simulink subsystem "PvtSubSys_LATC"  (R2020b)
settings: Solver=VariableStepAuto  StartTime=0.0  StopTime=10.0  RelTol=1e-3
undefined symbols (not defined in the file or in its folder): LCS_PLAN_PreViewIdxNum, LCS_PLAN_PreViewIdxSW_b, P_Global_CharSpd_ms, P_Global_SteeringAngleRatio, P_Global_WheelBase_m, P_LCS_DetNoOverRide_DrvTrq_TH, P_LCS_DetOverRide_DrvTrq_TH, P_LCS_ESS_AngleSlope_Limit, P_LCS_ESS_LogicTest_Enable, P_LCS_ESS_NotActiveFlgDelayTime, P_LCS_ESS_NotActiveFlgDelayTimeSW, P_LCS_ESS_SteerAngleErr, P_LCS_ESS_SteerAngleFilterTime, P_LCS_ESS_TarAngleFilterTime, P_LCS_ESSAngleSW, P_LCS_ESSOverrideTime1, P_LCS_ESSOverrideTime2, P_LCS_ESSOverrideTime3, P_LCS_ESSOverrideValue1, P_LCS_ESSOverrideValue2, P_LCS_IN_Offset_Test_SW, P_LCS_IN_Offset_Test_Value, P_LCS_LATC_AngleFilterTime_s, P_LCS_LATC_CurOffsetA2FliterT_s, P_LCS_LATC_CurOffsetCurve_TabX_m, P_LCS_LATC_CurOffsetCurveFliterTime_Tab_s, P_LCS_LATC_CurOffsetVehicleSpdLimitValue_degs, P_LCS_LATC_DeltaEps_Tab_s, P_LCS_LATC_DxOffset_Sw, P_LCS_LATC_ELKAngleSlope_ratio, P_LCS_LATC_ELKMaxLatAcc_ms2, P_LCS_LATC_ESSA0Dis_TabX_m, P_LCS_LATC_ESSAddAngleSlope_Tab_degs, P_LCS_LATC_ESSAESAngleSlope_Tab_degs, P_LCS_LATC_ESSAngleSlope_ratio, P_LCS_LATC_ESSMaxLatAcc_ms2, P_LCS_LATC_LCAngleSlope_ratio, P_LCS_LATC_LCAngleSlope_Tab_degs, P_LCS_LATC_LCCancleMaxLatAcc_ms2, P_LCS_LATC_LCEcoAngleSlope_ratio, P_LCS_LATC_LCEcoAngleSlope_Tab_degs, P_LCS_LATC_LCEcoMaxLatAcc_ms2, P_LCS_LATC_LCKAngleSlope_ratio, P_LCS_LATC_LCKAngleSlope_Tab_degs, P_LCS_LATC_LCKIEAngleSlope_ratio, P_LCS_LATC_LCKIEAngleSlope_Tab_degs, P_LCS_LATC_LCKIEMaxLatAcc_ms2, P_LCS_LATC_LCKMaxLatAcc_ms2, P_LCS_LATC_LCNormalAngleSlope_ratio, P_LCS_LATC_LCNormalAngleSlope_Tab_degs, P_LCS_LATC_LCNormalMaxLatAcc_ms2, P_LCS_LATC_LCSportAngleSlope_ratio, P_LCS_LATC_LCSportAngleSlope_Tab_degs, P_LCS_LATC_LCSportMaxLatAcc_ms2, P_LCS_LATC_LKAAngleSlope_ratio, P_LCS_LATC_LKAAngleSlope_Tab_degs, P_LCS_LATC_LKAMaxLatAcc_ms2, P_LCS_LATC_MatrixQ1_st, P_LCS_LATC_MatrixQ3_st, P_LCS_LATC_MatrixR_st ... (+77)
libraries: simulink x38
(part 6 of 7)

== matlab function PvtSubSys_LATC/LATC/LateralControl/LCS_Angle/Motion_Planning/CartesianTrajectory_MPC/CartesianTrajectory ==
  data: planX output single size=11; planY output single size=11; vEgo input size=1; planValid output boolean size=1; kapEgo input size=1; axEgo input size=1; TarLineValid input boolean size=1; TarLineC3 input size=1; TarLineC2 input size=1; TarLineC1 input size=1; TarLineC0 input size=1; ayDtLimit input size=1; planT output; LoopNum output; planLength output; Ay output size=11; AyDt output size=11; break_Flg output; break_AyValue output; break_AyDtValue output; PreDis input; Dis_Fac input; Min_PlanDis input
function [planX,planY,planValid,planT,LoopNum,planLength,Ay,AyDt,break_Flg,break_AyValue,break_AyDtValue] = ...
    linePlanCalc(vEgo, kapEgo,axEgo,...
    TarLineValid,TarLineC3,TarLineC2,TarLineC1,TarLineC0,...
    ayDtLimit,PreDis,Dis_Fac,Min_PlanDis)
%五次多项式规划
LoopNum = 0;
if TarLineValid
    if (abs(TarLineC0)<single(0)) && (abs(TarLineC1)<single(0.05))  %控制线不走中心线，走规划线
        planValid = true;
        planT = single(11);
        planX = single(zeros(11,1));
        planY = single(zeros(11,1));
        planX = single((linspace(0,40,11)))';
        planY = TarLineC3.*planX.^3 + TarLineC2.*planX.^2 + TarLineC1*planX + TarLineC0;
        planLength = planX(end,1);
        Ay = single(zeros(11,1));
        AyDt = single(zeros(11,1));
        break_Flg = uint8(0);
        break_AyValue = single(0);
        break_AyDtValue = single(0);
    else
        Px =single([1.4 1.6 2.1 2.3 2.5 2.7 3 3.3 3.6 4 4.4 4.8 5.3 5.8 6.4 7.1 7.8 8.6 9.5 10.4 11.4]);% 按等比1.1  初选规划时间
        % 定义 TarEgoV、TarEgoAx，由于时间点数变化，导致轨迹条数变化，因此TarEgoV、TarEgoAx维数需要重新定义
        TarEgoAx = zeros(1,length(Px));
        TarEgoV = ones(1,length(Px)) .* vEgo;
        
        if vEgo>single(1)
            Px = vEgo*Px;   %纵向行驶距离
        end
        
        Py = TarLineC3*(Px.^3) + TarLineC2*(Px.^2) + TarLineC1*(Px.^1) + TarLineC0;
        x = single(zeros(11,1));
        y = single(zeros(11,1));
        Vx = single(zeros(11,1));
        Vy = single(zeros(11,1));
        Ax = single(zeros(11,1));
        Ay = single(zeros(11,1));
        AyDt = single(zeros(11,1));
        
        break_Flg = uint8(0);
        break_AyValue = single(0);
        break_AyDtValue = single(0);

        Pt = single(zeros(1,1));  
        for i = 1:length(Px)   
            Pt = 1.05*sqrt(Px(i)^2 + Py(i)^2)/max(1,0.5*(TarEgoV(i) + vEgo));  %规划时间
            t_Vego = max(vEgo,1);
            t0 = single(0);
            tn = Pt;
            
            T = [t0^5,t0^4,t0^3,t0^2,t0,1;...
                5*t0^4,4*t0^3,3*t0^2,2*t0,1,0;...
                20*t0^3,12*t0^2,6*t0,2,0,0;...
                tn^5,tn^4,tn^3,tn^2,tn,1;...
                5*tn^4,4*tn^3,3*tn^2,2*tn,1,0;...
                20*tn^3,12*tn^2,6*tn,2,0,0];    
            
            Vn = TarEgoV(i);
            An = TarEgoAx(i);
            kP =  3*TarLineC3*(Px(i).^2) + 2*TarLineC2*Px(i) + TarLineC1;  %规划线的斜率
            
            Kap = 6*TarLineC3*(Px(i))+2*TarLineC2;      
            Arcf = (vEgo^2)*Kap;                          
            Ayn = Arcf/sqrt(1 + kP^2);                       
            Axn = Arcf*kP/sqrt(1 + kP^2);                              
            Vxn = Vn/sqrt(1 + kP^2);                         
            Vyn = Vn*kP/sqrt(1 + kP^2);
            
            MaX = [0;t_Vego;axEgo;Px(i);Vxn;Axn];            
            MaY = [0;0;(vEgo^2)*kapEgo;Py(i);Vyn;Ayn];
            %求解多项式
            A = T\MaX;
            B = T\MaY;
            
            a5 = A(1);
            a4 = A(2);
            a3 = A(3);
            a2 = A(4);
            a1 = A(5);
            a0 = A(6);
            
            b5 = B(1);
            b4 = B(2);
            b3 = B(3);
            b2 = B(4);
            b1 = B(5);
            b0 = B(6);
            
            preLineValid = true;
            for j=1:11
                t = (j-1)*tn/10;
                x(j) = a5*t^5 + a4*t^4 + a3*t^3 + a2*t^2 + a1*t + a0;
                Vx(j) = 5*a5*t^4 + 4*a4*t^3 + 3*a3*t^2 + 2*a2*t + a1;
                Ax(j) = 20*a5*t^3 + 12*a4*t^2 + 6*a3*t + 2*a2;
                y(j) = b5*t^5 + b4*t^4 + b3*t^3 + b2*t^2 + b1*t + b0;
                Vy(j) = 5*b5*t^4 + 4*b4*t^3 + 3*b3*t^2 + 2*b2*t + b1;
                Ay(j) = 20*b5*t^3 + 12*b4*t^2 + 6*b3*t + 2*b2;
                AyDt(j) = 60*b5*t^2 + 24*b4*t + 6*b3;

                if (abs(AyDt(j))>ayDtLimit)
                    break_Flg = uint8(1);
                    break_AyValue = abs(Ay(j));
                    break_AyDtValue = abs(AyDt(j));
                    preLineValid = false;
                    break;
                end
            end
            if ((sqrt(x(11)^2 + y(11)^2)) < Min_PlanDis) || ((sqrt(x(11)^2 + y(11)^2))*Dis_Fac < (PreDis + 2.1))
                preLineValid = false;
            end
            if preLineValid
                break_Flg = uint8(3);
                break_AyValue = max(abs(Ay));
                break_AyDtValue = max(abs(AyDt(j)));
                break;
            end
            
            if i == length(Px) % 此处存在都不满足的情况，需要按最长时间输出。经测试发现如果按最长时间输出会控不住车辆。暂时改成跟随目标线
                planValid = true;
                Pt = single(Px(i));
                x = single(zeros(11,1));
                y = single(zeros(11,1));
                x = single((linspace(0,40,11)))';
                y = TarLineC3.*x.^3 + TarLineC2.*x.^2 + TarLineC1*x + TarLineC0;
                break_Flg = uint8(4);
                break_AyValue = single(0);
                break_AyDtValue = single(0);
            end
        end
        LoopNum = i;
        planValid = true;
        planT = Pt;
        planX = x;
        planY = y;
        planLength = planX(end,1);
    end
else
    planValid = false;
    planT = single(0);
    planX = single(zeros(11,1));
    planY = single(zeros(11,1));
    LoopNum = 0;
    planLength = planX(end,1);
    Ay = single(zeros(11,1));
    AyDt = single(zeros(11,1));
    break_Flg = uint8(0);
    break_AyValue = single(0);
    break_AyDtValue = single(0);
end

== matlab function PvtSubSys_LATC/LATC/LateralControl/LCS_Angle/Motion_Planning/FrenetTrajectory/Subsystem/MATLAB Function1 ==
  data: Delaytime input uint16; Flg output uint8; Count output uint16; TarDangerLevel input uint8; TarDangerLevelK1 input uint8; FlgK1 input uint8; CountK1 input uint16
function [Flg,Count]= fcn(Delaytime,TarDangerLevel,TarDangerLevelK1,FlgK1,CountK1)
Count = min(CountK1 + uint16(1),Delaytime);
if Count == Delaytime
    Flg = uint8(0);
else
    Flg = FlgK1;
end
%%状态检测
if TarDangerLevel == uint8(1) && TarDangerLevelK1 == 0 %功能激活
    Count = uint16(0);
    Flg = uint8(1);  
end
end

== matlab function PvtSubSys_LATC/LATC/LateralControl/EPSFaultCheck/MATLAB Function1 ==
  data: u input; y output uint8; countK input uint8; count output uint8
function [y,count] = fcn(u,countK)
count = countK - uint8(1);
if u>0
    count = uint8(3000);
end
if count > 1
    y = uint8(0);
else
    y = uint8(1);
end

== matlab function PvtSubSys_LATC/LATC/LateralControl/LCS_Angle/Lateral_Control/Dynamic_Model_LQR/TarSteerAngleCalc ==
  data: steer_angle_cmd_temp output; steer_feedforward_temp output; steer_feedbackward_temp output; steer_limit_temp output; LineValid input; SteerAngle input; steer_angle output size=[1,1]; Veh_Speed input; ref_curvature input; lateral_error input; lateral_error_rate input; heading_error input; heading_error_rate input; Left_steer_ratio input; Right_steer_ratio input; Matrix_q1 input; Matrix_q3 input; Matrix_R input; Max_lateral_acceleration input; TarSteerAngleSlope input; CurrentSteerAngleOffset input; steer_angleK1 input single
function [steer_angle_cmd_temp,steer_feedforward_temp,steer_feedbackward_temp,steer_limit_temp,steer_angle]= LQR_Algorithm(LineValid,SteerAngle,Veh_Speed,ref_curvature,lateral_error,lateral_error_rate,heading_error,heading_error_rate,...
    Left_steer_ratio,Right_steer_ratio,Matrix_q1,Matrix_q3,Matrix_R,Max_lateral_acceleration,TarSteerAngleSlope,CurrentSteerAngleOffset,steer_angleK1)
if LineValid
    %% 1.车辆参数
    %1.1 车的大小及长度参数
    veh_params.vehicle_length = single(4.875);
    veh_params.vehicle_width  = single(2.2);
    veh_params.vehicle_height = single(1.69);
    %1.2 车辆控制参数
    veh_params.wheel_base = single(2.92);               %轴距, m
    veh_params.Vch = single(23.5);                      %特征车速
    veh_params.max_steer_angle = single(53 / 180 * pi); %前轮最大转角
    veh_params.max_acceleration = single(2);            %车辆最大加速度
    veh_params.max_deceleration = single(-2);           %车辆最大减速度
    veh_params.left_steer_ratio = Left_steer_ratio;     %车辆左侧转向传动比%
    veh_params.right_steer_ratio = Right_steer_ratio;   %车辆右侧转向传动比%
    veh_params.cf = single(155494.663);                 %车辆前轮侧偏刚度
    veh_params.cr = single(155494.663);                 %车辆后轮侧偏刚度 
    veh_params.mass_fl = single(520);                   %车辆左前轮负重
    veh_params.mass_fr = single(520);                   %车辆右前轮负重
    veh_params.mass_rl = single(520);                   %车辆左后轮负重
    veh_params.mass_rr = single(520);                   %车辆右后轮负重
    %% 2.控制参数计算
    mass_front =  veh_params.mass_fl + veh_params.mass_fr;     %前轮负载
    mass_rear  =  veh_params.mass_rl + veh_params.mass_rr;     %后轮负载
    mass =  mass_front + mass_rear;                            %这个整车负载  不是整车质量？？？？？？？
    lf = veh_params.wheel_base * (single(1.0) - mass_front / mass);
    lr = veh_params.wheel_base * (single(1.0) - mass_rear / mass);
    iz = lf * lf * mass_front + lr * lr * mass_rear;
    %% 3.LQR参数设置
    
    lqr_eps = single(0.01);    %最小精度
    lqr_max_iteration = single(800);    %最大迭代次数
    
    basic_state_size = uint8(4);     
    control_size = uint8(1);
    
    matrix_a = single(zeros(basic_state_size,basic_state_size));
    matrix_a_coeff = single(zeros(basic_state_size,basic_state_size));
    I = single(eye(basic_state_size,basic_state_size));
    matrix_a(1,2) = single(1.0);
    matrix_a(2,3) = single((veh_params.cf + veh_params.cr ) / mass);
    matrix_a(3,4) = single(1.0);
    matrix_a(4,3) = single((lf * veh_params.cf - lr * veh_params.cr) / iz);
    
    matrix_a_coeff(2,2) = single(-(veh_params.cf + veh_params.cr) / mass);
    matrix_a_coeff(2,4) = single((lr * veh_params.cr - lf * veh_params.cf) / mass);
    matrix_a_coeff(3,4) = single(1.0);
    matrix_a_coeff(4,2) = single((lr * veh_params.cr - lf * veh_params.cf) / iz);
    matrix_a_coeff(4,4) = single(-1.0 * (lf * lf * veh_params.cf + lr * lr * veh_params.cr)/iz);
    
    matrix_a(2,2) = matrix_a_coeff(2,2);
    matrix_a(2,4) = matrix_a_coeff(2,4);
    matrix_a(4,2) = matrix_a_coeff(4,2);
    matrix_a(4,4) = matrix_a_coeff(4,4);
    
    matrix_b = single(zeros(basic_state_size,control_size));
    matrix_b(2,1) = veh_params.cf/mass;
    matrix_b(4,1) = lf * veh_params.cf /iz;
    
    matrix_q = single(zeros(4,4));
    matrix_q(1,1) = Matrix_q1;                      %调整q矩阵的第一、三个参数，改善转向性能0.0001,0.02  Q为状态权重系数
    matrix_q(3,3) = Matrix_q3;
    matrix_r = single(zeros(1,1));
    matrix_r = Matrix_R;                            %R为控制量权重系数
    
    lqr_params.A = matrix_a;
    lqr_params.B = matrix_b;
    lqr_params.I = I;
    lqr_params.ts = single(0.02);
    lqr_params.lr = lr;
    lqr_params.lf = lf;
    lqr_params.cf=veh_params.cf;
    lqr_params.cr=veh_params.cf;
    lqr_params.iz=iz;
    lqr_params.mass=mass;
    lqr_params.Q =matrix_q ;
    lqr_params.R = matrix_r;
    lqr_params.eps=lqr_eps;
    lqr_params.max_iteration=lqr_max_iteration;
    %% 4.计算前轮转角
    lqr_params.A(2,2) = lqr_params.A(2,2)/(max(Veh_Speed, single(0.2)));
    lqr_params.A(2,4) = lqr_params.A(2,4)/(max(Veh_Speed, single(0.2)));
    lqr_params.A(4,2) = lqr_params.A(4,2)/(max(Veh_Speed, single(0.2)));
    lqr_params.A(4,4) = lqr_params.A(4,4)/(max(Veh_Speed, single(0.2)));
    
    A=lqr_params.A;
    B=lqr_params.B;
    I=lqr_params.I;
    ts=lqr_params.ts;      %控制周期
    min_tol = lqr_params.eps;    %0.01  这个时间是什么意思？？？？？？
    max_iter = lqr_params.max_iteration;   %800   这个是什么意思？？？？？
    matrix_Q = lqr_params.Q;
    matrix_R = lqr_params.R;
    
    matrix_ad=single(zeros(size(A)));   %4*4零矩阵
    matrix_ad=(I+ts*single(0.5) * A) / (I-ts*single(0.5) * A);  %离散化 系数 A=(I-TA/2)/(I-TA/2) B=TB
    
    matrix_bd=single(zeros(size(B)));
    matrix_bd=B*ts;
    matrix_k = SolveLQRProblem(matrix_ad, matrix_bd, matrix_Q,matrix_R, min_tol, max_iter);  %求解最优解K
    %% 横向状态变量
    
    matrix_state = single(zeros(4, 1));
    matrix_state(1, 1) = lateral_error;                   %横向误差
    matrix_state(2, 1) = lateral_error_rate;              %横向误差率
    matrix_state(3, 1) = heading_error;                   %航向误差
    matrix_state(4, 1) = heading_error_rate;              %航向误差率
    steer_feedbackward = -(matrix_k * matrix_state);      %反馈控制器
    % 前馈转角
    kv = lqr_params.lr * lqr_params.mass / single(1) / lqr_params.cf / veh_params.wheel_base - ...
        lqr_params.lf * lqr_params.mass / single(1) / lqr_params.cr / veh_params.wheel_base;
    steer_feedforward = (veh_params.wheel_base * ref_curvature + kv * Veh_Speed * Veh_Speed * ref_curvature - matrix_k(1, 3) * ...
        (lqr_params.lr * ref_curvature - lqr_params.lf * lqr_params.mass * Veh_Speed * Veh_Speed * ref_curvature / single(1) / lqr_params.cr / veh_params.wheel_base));%弧度制角度rad
    % 4.3 计算期望前轮偏角
    steer_cmd = steer_feedforward + steer_feedbackward;
    
    if (steer_cmd>=0)
        steer_transmission_ratio = veh_params.left_steer_ratio;
    else
        steer_transmission_ratio = veh_params.right_steer_ratio;
    end
    steer_feedforward_temp = steer_feedforward * single(57.3) * steer_transmission_ratio;%反算方向盘转角并转换为角度制deg
    steer_feedbackward_temp = steer_feedbackward * single(57.3) * steer_transmission_ratio;%反算方向盘转角并转换为角度制deg
    steer_angle_cmd = steer_cmd * single(57.3) * steer_transmission_ratio;%反算方向盘转角并转换为角度制deg
    steer_angle_cmd_temp = steer_angle_cmd;%输出算法计算角度作为观测，最终请求角度会补偿转向不足。
    %% 5.限制期望前轮偏角
    % 5.1 根据横向加速度限制前轮转角
    if Veh_Speed < 1
        steer_limit = atan( Max_lateral_acceleration * veh_params.wheel_base /(Veh_Speed *Veh_Speed))* single(57.3) * steer_transmission_ratio; % 高速计算不准确，更改为下面特征车速计算方法
    else
        AckConst = min((single(1)+Veh_Speed*Veh_Speed/(veh_params.Vch*veh_params.Vch))*veh_params.wheel_base/max(single(1),Veh_Speed),single(32767));
        % PsiDtAckRaw = (SteerAngle/steer_transmission_ratio)/AckConst;
        steer_limit = ((Max_lateral_acceleration * AckConst)/Veh_Speed)* single(57.3) * steer_transmission_ratio;
    end
    %     steer_limit = atan( Max_lateral_acceleration * veh_params.wheel_base /(Veh_Speed *Veh_Speed)) * steer_transmission_ratio;
    steer_angle_cmd = min(steer_limit, max(-steer_limit,steer_angle_cmd));%方向盘角度制deg
    
    steer_angle_deg = steer_angle_cmd + CurrentSteerAngleOffset;
    steer_limit_temp = steer_limit;
    % 5.2 限制方向盘转速
    steer_angle = min(steer_angleK1 + TarSteerAngleSlope,max(steer_angleK1 - TarSteerAngleSlope,steer_angle_deg));
    
else
    steer_angle = SteerAngle;
    steer_angle_cmd_temp = single(0);
    steer_feedforward_temp = single(0);
    steer_feedbackward_temp = single(0);
    steer_limit_temp = single(0);
end
end

== matlab function PvtSubSys_LATC/LATC/LateralControl/LCS_Angle/Motion_Planning/CartesianTrajectory/Subsystem1/MATLAB Function ==
  data: Forward_PreViewT input; VehSpd input; PreCurve output; C2 input; C3 input; PreCurve_Abs output
function [PreCurve,PreCurve_Abs]= PreView_Point_Curvature(Forward_PreViewT,VehSpd,C2,C3)
LookForwardDis = VehSpd * Forward_PreViewT;
PreCurve = 6*C3*LookForwardDis + 2*C2;
PreCurve_Abs = abs(PreCurve);
end

== matlab function PvtSubSys_LATC/LATC/LateralControl/LCS_Angle/Motion_Planning/CartesianTrajectory/Subsystem1/MATLAB Function1 ==
  data: Delaytime input uint16; Flg output uint8; Count output uint16; TarDangerLevel input uint8; TarDangerLevelK1 input uint8; FlgK1 input uint8; CountK1 input uint16
function [Flg,Count]= fcn(Delaytime,TarDangerLevel,TarDangerLevelK1,FlgK1,CountK1)
Count = min(CountK1 + uint16(1),Delaytime);
if Count == Delaytime
    Flg = uint8(0);
else
    Flg = FlgK1;
end
%%状态检测
if TarDangerLevel == uint8(1) && TarDangerLevelK1 == 0 %功能激活
    Count = uint16(0);
    Flg = uint8(1);  
end
end

== matlab function PvtSubSys_LATC/LATC/LateralControl/LCS_Angle/Motion_Planning/CartesianTrajectory/FrenetTrajectory ==
  data: A0 input; A1 input; A2 input; A3 input; Veh_Speed input size=1; YawRate input size=1; PreView_T input size=1; PlanX output; PlanY output; PlanTheta output; idx output; PreviewX output; PreviewY output; PreviewTheta output; numTraj output size=1; ref_curvature output; ref_theta output; AyDtLimit input size=1; Min_Plan_Dis input; lateral_error output size=1; lateral_error_rate output size=1; heading_error output size=1; heading_error_rate output size=1; axEgo input; kapEgo input; PreViewIdxSW input size=[1,1]; PreViewIdxNum input size=[1,1]
function [PlanX,PlanY,PlanTheta,idx,PreviewX,PreviewY,PreviewTheta,numTraj,ref_curvature,ref_theta,lateral_error,lateral_error_rate,heading_error,heading_error_rate] ...
    = FrenetTrajectory(A0,A1,A2,A3,Veh_Speed,YawRate,PreView_T,AyDtLimit,Min_Plan_Dis,axEgo,kapEgo,PreViewIdxSW,PreViewIdxNum)
%% 生成轨迹
Px =single([1.5 2 2.5 2.7 3 3.3 3.6 4 4.4 4.8 5.3 5.8 6.4 7.1 7.8 8.6 9.5 10.4 11.4]); %Py_Fac后期去掉，增加一个轨迹筛选条件，每个车速下最小规划距离
TarEgoAx = zeros(1,length(Px));   %初始化矩阵
TarEgoV = ones(1,length(Px)) .* Veh_Speed;  %计算纵向行驶距离
if Veh_Speed>single(1)
    Px = Veh_Speed*Px;    %纵向距离 l 
end 
Py = A3*(Px.^3) + A2*(Px.^2) + A1*(Px.^1) + A0;  
x = single(zeros(11,1));
y = single(zeros(11,1));
Vx = single(zeros(11,1));
Vy = single(zeros(11,1));
Ax = single(zeros(11,1));
Ay = single(zeros(11,1));
AyDt = single(zeros(11,1));
Pt = single(zeros(1,1));     %规划时间
for i = 1:length(Py)
    Pt = 1.05*sqrt(Px(i)^2 + Py(i)^2)/max(1,0.5*(TarEgoV(i) + Veh_Speed));   
    t_Vego = max(Veh_Speed,1);
    t0 = single(0);
    tn = Pt;
    T = [t0^5,t0^4,t0^3,t0^2,t0,1;...
        5*t0^4,4*t0^3,3*t0^2,2*t0,1,0;...
        20*t0^3,12*t0^2,6*t0,2,0,0;...
        tn^5,tn^4,tn^3,tn^2,tn,1;...
        5*tn^4,4*tn^3,3*tn^2,2*tn,1,0;...
        20*tn^3,12*tn^2,6*tn,2,0,0];
    Vn = TarEgoV(i);
    An = TarEgoAx(i);
    kP =  3*A3*(Px(i).^2) + 2*A2*Px(i) + A1;
    
    Kap = 6*A3*(Px(i))+2*A2;
    Arcf = (Veh_Speed^2)*Kap;
    Ayn = Arcf/sqrt(1 + kP^2);
    Axn = Arcf*kP/sqrt(1 + kP^2);
    
    Vxn = Vn/sqrt(1 + kP^2);
    Vyn = Vn*kP/sqrt(1 + kP^2);
    MaX = [0;t_Vego;axEgo;Px(i);Vxn;Axn];
    MaY = [0;0;(Veh_Speed^2)*kapEgo;Py(i);Vyn;Ayn];
    A = T\MaX;
    B = T\MaY;
    
    a5 = A(1); % 纵向轨迹系数
    a4 = A(2);
    a3 = A(3);
    a2 = A(4);
    a1 = A(5);
    a0 = A(6);
    
    b5 = B(1); % 横向轨迹系数
    b4 = B(2);
    b3 = B(3);
    b2 = B(4);
    b1 = B(5);
    b0 = B(6);
    preLineValid = true;
    for j=1:11
        t = (j-1)*tn/10;
        x(j) = a5*t^5 + a4*t^4 + a3*t^3 + a2*t^2 + a1*t + a0;
        Vx(j) = 5*a5*t^4 + 4*a4*t^3 + 3*a3*t^2 + 2*a2*t + a1;
        Ax(j) = 20*a5*t^3 + 12*a4*t^2 + 6*a3*t + 2*a2;
        y(j) = b5*t^5 + b4*t^4 + b3*t^3 + b2*t^2 + b1*t + b0;
        Vy(j) = 5*b5*t^4 + 4*b4*t^3 + 3*b3*t^2 + 2*b2*t + b1;
        Ay(j) = 20*b5*t^3 + 12*b4*t^2 + 6*b3*t + 2*b2;
        AyDt(j) = 60*b5*t^2 + 24*b4*t + 6*b3;
        if abs(AyDt(j))>AyDtLimit 
            preLineValid = false;
            break;
        end     
    end
    if abs(sqrt(x(11)^2+y(11)^2)) < Min_Plan_Dis       %规划的距离最小不能小于设定的阈值
       preLineValid = false; 
    end
    if preLineValid
        break;
    end
end
NumTarpoints = 40;       %轨迹点的个数
y = y.*single(-1);
objSpline = Spline2D(y,x);
s = single(linspace(0,objSpline.s(end),NumTarpoints));
TargetPoints = single(zeros(length(s),6));
%% 为什么要转一下直角坐标？？？？？

for i = single(1):single(1):length(s)
    [ix,iy] = objSpline.calc_position(s(i));     %车体坐标转换为直角坐标
    TargetPoints(i,1) = ix;                      %直角坐标中的X 左负右正   车辆横向位置
    TargetPoints(i,2) = iy;                      %直角坐标Y    车辆纵向位置
    TargetPoints(i,3) = objSpline.calc_yaw(s(i));   %车辆Yaw角  横摆角
    TargetPoints(i,4) = objSpline.calc_curvature(s(i));    %曲率
    TargetPoints(i,5) = objSpline.calc_curvatureDerivative(s(i));   %曲率变化率
    TargetPoints(i,6) = s(i);                                  
end
traj = single(zeros(NumTarpoints,6)); t= single(zeros(NumTarpoints,1)); costs = single(zeros(1,1));
globalTrajectory = repmat(struct('Trajectory',traj,'Times',t,'costs',costs), 1, 1);
globalTrajectory(1).Trajectory = TargetPoints;
globalTrajectory(1).Times = t;

numTraj  = i;%借用numTraj输出时间点索引号
%% 直角坐标转换为车体坐标     
% [s,d]→[x, y, theta, kappa, dkappa]
PlanX= globalTrajectory(1).Trajectory(1:NumTarpoints,2);
PlanY= (globalTrajectory(1).Trajectory(1:NumTarpoints,1))*single(-1);
PlanTheta = globalTrajectory(1).Trajectory(1:NumTarpoints,3);
[matrix_state,ref_curvature,ref_theta,idx] = Calc_State_Error(Veh_Speed,YawRate,globalTrajectory,PreView_T,NumTarpoints,PreViewIdxSW,PreViewIdxNum);
PreviewX = globalTrajectory(1).Trajectory(idx,2);
PreviewY = (globalTrajectory(1).Trajectory(idx,1))*single(-1);
PreviewTheta = globalTrajectory(1).Trajectory(idx,3);
% lateral_error = single(zeros(1,1));lateral_error_rate = single(zeros(1,1));heading_error = single(zeros(1,1));heading_error_rate = single(zeros(1,1));
lateral_error = matrix_state(1,1);
lateral_error_rate = matrix_state(2,1);
heading_error = matrix_state(3,1);
heading_error_rate = matrix_state(4,1);

end

== matlab function PvtSubSys_LATC/LATC/LateralControl/ESS_SteerSpd_Test/NotActiveFlgDelayTime/MATLAB Function ==
  data: FlgIn input boolean; FlgOut output boolean size=1; t_offset input single; tcycle input single; FlgOutK1 input boolean; delaytimeK1 input single; delaytime output single size=1; flgK1 input uint8; flg output uint8 size=1
function [FlgOut,delaytime,flg]= fcn(FlgIn,t_offset,tcycle,FlgOutK1,delaytimeK1,flgK1)
FlgOut = FlgIn;
delaytime = single(0);
flg = uint8(0);
if FlgOutK1 ==0 && FlgOut == 1
    flg = uint8(1);
    FlgOut = true;
    delaytime = tcycle;
end
if  flgK1 == 1
     delaytime = delaytimeK1 + tcycle;
      if delaytime < t_offset
          flg = uint8(1);
          FlgOut = true;
      end
end

== matlab function PvtSubSys_LATC/LATC/LateralControl/LCS_Angle/Lateral_Control/kinematics_MPC/SteerAngSlopeCalc/MATLAB Function3 ==
  data: delytime input uint16; TarDangerLevel input uint8; TarDangerLevelK1 input uint8; FLg output uint8; FLgK1 input uint8; CntK1 input uint16; Cnt output uint16
function [FLg,Cnt] = AngSlopeCalc(delytime,TarDangerLevel,TarDangerLevelK1,FLgK1,CntK1)

Cnt = min(CntK1 + uint16(1),delytime);
if Cnt== delytime
    FLg = uint8(0);
else
    FLg = FLgK1;
end
%FLg = FLgK1;
%% 
if TarDangerLevel==uint8(1) && TarDangerLevelK1==0  % NO function 2 LCK (TarDangerLevelK1==0)
    Cnt =uint16(0);
    FLg = uint8(1);
end

if  TarDangerLevel==uint8(3) && (TarDangerLevelK1==uint8(1)||TarDangerLevelK1==uint8(2)) % LCK/IE 2 LC_Normal
    Cnt =uint16(0);
    FLg = uint8(2);
end

if  TarDangerLevel==uint8(7) && (TarDangerLevelK1==uint8(1)||TarDangerLevelK1==uint8(2)) % LCK/IE 2 LC_Eco
    Cnt =uint16(0);
    FLg = uint8(3);
end

if  TarDangerLevel==uint8(8) && (TarDangerLevelK1==uint8(1)||TarDangerLevelK1==uint8(2)) % LCK/IE 2 LC_sport
    Cnt =uint16(0);
    FLg = uint8(4);
end
if  TarDangerLevel==uint8(6) && (TarDangerLevelK1==uint8(1)||TarDangerLevelK1==uint8(2)) % LCK/IE 2 ESS 后期添加配和ESS Slope 一起调试
    Cnt =uint16(0);
    FLg = uint8(5);
end

== matlab function PvtSubSys_LATC/LATC/LateralControl/LCS_Angle/Lateral_Control/kinematics_MPC/TarSteerAngleCalc ==
  data: steer_angle_cmd_temp output; steer_feedforward_temp output; steer_feedbackward_temp output; steer_limit_temp output; matrix_result output; LineValid input; SteerAngle input; steer_angle output size=[1,1]; Veh_Speed input; ref_curve input; ref_theta input; Delta_t input; lateral_error input; heading_error input; Umax input; Delta_umax input; Left_steer_ratio input; Right_steer_ratio input; Matrix_q1 input; Matrix_q2 input; Matrix_r input; Max_lateral_acceleration input; TarSteerAngleSlope input; CurrentSteerAngleOffset input; steer_angleK1 input single; U_k output; U_k1 input single
function [steer_angle_cmd_temp,steer_feedforward_temp,steer_feedbackward_temp,steer_limit_temp,matrix_result,steer_angle,U_k]= ...
    kinematics_MPC(LineValid,SteerAngle,Veh_Speed,ref_curve,ref_theta,Delta_t,lateral_error,heading_error,Umax,Delta_umax,...
    Left_steer_ratio,Right_steer_ratio,Matrix_q1,Matrix_q2,Matrix_r,Max_lateral_acceleration,TarSteerAngleSlope,CurrentSteerAngleOffset,steer_angleK1,U_k1)
if LineValid
    %% 1.车辆参数
    %1.1 车的大小及长度参数
    veh_params.vehicle_length = single(4.875);
    veh_params.vehicle_width  = single(2.2);
    veh_params.vehicle_height = single(1.69);
    %1.2 车辆控制参数
    veh_params.wheel_base = single(2.92);               %轴距, m
    veh_params.Vch = single(23.5);                      %特征车速
    veh_params.max_steer_angle = single(53 / 180 * pi); %前轮最大转角  
    veh_params.max_acceleration = single(2);            %车辆最大加速度
    veh_params.max_deceleration = single(-2);           %车辆最大减速度
    veh_params.left_steer_ratio = Left_steer_ratio;     %车辆左侧转向传动比%
    veh_params.right_steer_ratio = Right_steer_ratio;   %车辆右侧转向传动比%
    veh_params.cf = single(155494.663);                 %车辆前轮侧偏刚度
    veh_params.cr = single(155494.663);                 %车辆后轮侧偏刚度 
    veh_params.mass_fl = single(520);                   %车辆左前轮负重
    veh_params.mass_fr = single(520);                   %车辆右前轮负重
    veh_params.mass_rl = single(520);                   %车辆左后轮负重
    veh_params.mass_rr = single(520);                   %车辆右后轮负重
    %% 2.控制参数计算
    %% 3.MPC矩阵
    Np = single(10);
    Nc = single(5);
    Row = single(10); %松弛因子
    ref_delta = atan(veh_params.wheel_base * ref_curve);   %前轮转角
    %% 离散状态空间方程
    A = [ 1  Veh_Speed * cos(ref_theta) * Delta_t;    %一个是航向角一个是前轮转角  这里都用前轮转角对吗？
        0  1 ];
    B = [ 0;
        Veh_Speed * Delta_t / (veh_params.wheel_base * cos(ref_delta)^2)];
    Nx = size(A,1); %状态量个数 2 横向车速V及航向角
    Nu = size(B,2); %控制量个数 1 前轮转角
    % 对状态量进行增广
    kesi = zeros(Nx,Nu); % 构造新的状态量矩阵   2*1
    kesi = cat(1,kesi,U_k1);% 将上一时刻的前轮偏角误差放在第3行，进行状态增广3*1维矩阵
    kesi(1) = lateral_error;
    kesi(2) = lateral_error;  %即kesi矩阵为[lateral_error;lateral_error;ref_delta_error]
    %% 定义Q R矩阵
    matrix_q = [Matrix_q1 0;
                0 Matrix_q2];
    matrix_r = Matrix_r;
    matrix_Q = zeros(Np*Nx,Np*Nx);%20*20
    matrix_Q_temp = zeros(Nx,Np*Nx);%2*20
    for i=1:Np
        for j= 1:Np
            if i == j
                matrix_Q_temp = zeros(Nx,Np*Nx);
                matrix_Q_temp(:,((j-1)*Nx+1):j*Nx) = matrix_q;
            end
        end
        matrix_Q(((i-1)*Nx+1):i*Nx,:) = matrix_Q_temp;
    end
    matrix_R = zeros(Nc*Nu,Nc*Nu);%10*10
    matrix_R_temp = zeros(Nu,Nc*Nu);
    for i=1:Nc
        for j= 1:Nc
            if i == j
                matrix_R_temp = zeros(Nu,Nc*Nu);
                matrix_R_temp(:,((j-1)*Nu+1):j*Nu) = matrix_r;
            end
        end
        matrix_R(((i-1)*Nu+1):i*Nu,:) = matrix_R_temp;
    end
    % 按增量式对矩阵进行增广
    A = [A B;zeros(Nu,Nx) eye(Nu)]; % 3*3
    B = [B;eye(Nu)]; % 3*1
    % 定义输出矩阵
    C = single([1 0 0;0 1 0;]);% 2*3
    % THETA和PHI
    PHI = zeros(Np*Nx,size(A,2));    %20*3
    THETA = zeros(Np*Nx,Nc*Nu);      %20*5
    THETA_temp = zeros(Nx,Nc*Nu);    %2*5
    for r=1:Np
        for c=1:Nc
            if c<=r
                THETA_temp(:,((c-1)*Nu+1):c*Nu)=C*A^(r-c)*B; %2*3*3*3*1
            end
        end
        THETA(((r-1)*Nx+1):r*Nx,:) = THETA_temp;
        PHI(((r-1)*Nx+1):r*Nx,:) =  C*A^r; %2*3*3*3
    end
    
    % 构造二次规划的H矩阵
    H_temp = THETA'*matrix_Q*THETA + matrix_R;
    H = [H_temp zeros(Nu*Nc,1);zeros(1,Nu*Nc) Row];
    H = single(2)*H;
    H = (H+H')/single(2);
    % E矩阵
    error = PHI*kesi; %这里的error就是我们所设的E矩阵
    % f矩阵
    f_temp = single(2)*error'* matrix_Q * THETA;
    f = zeros(size(f_temp,1),(size(f_temp,2)+1));
    f(:,1:size(f_temp,2)) = f_temp;
    %% 约束生成区域
    % 不等式约束
    A_t = tril(ones(Nc,Nc),0);
    A_I=kron(A_t,eye(Nu));
    Ut=kron(ones(Nc,1),U_k1);                 %此处的U表示的应该是上一时刻控制量误差（即偏差）组成的矩阵。
    umin = -Umax/single(57.3);                %维数与控制变量的个数相同
    umax = Umax/single(57.3);                 %此处的最大值最小值约束，是对控制量误差的最大最小值进行约束，此处理解的物理意义是在参考转角上下一个范围内进行约束求解
    
    delta_umin =  -Delta_umax/single(57.3)*Delta_t;
    delta_umax =   Delta_umax/single(57.3)*Delta_t;
    Umin=kron(ones(Nc,1),umin);
    Umax=kron(ones(Nc,1),umax);
%     A_cons = [A_I zeros(Nu*Nc,1);-A_I zeros(Nu*Nc,1)];
%     b_cons = [Umax-Ut;-Umin+Ut];
    % 上下限约束
    EM = single(10);
    delta_Umin=kron(ones(Nc,1),delta_umin);
    delta_Umax=kron(ones(Nc,1),delta_umax);
    lb=[delta_Umin;-EM];%（求解方程）状态量下界，包含控制时域内控制增量和松弛因子下界M
    ub=[delta_Umax;EM];%（求解方程）状态量上界，包含控制时域内控制增量和松弛因子上界M
    % 两种约束合并
    A_cons2 = [A_I zeros(Nu*Nc,1);-A_I zeros(Nu*Nc,1);eye((Nu*Nc)+1);-eye((Nu*Nc)+1)];
    b_cons2 = [Umax-Ut;-Umin+Ut;ub;-lb];
    %% 二次规划求解
    % Format in qp_solver
    % min 0.5*x'*H*x + f'*x   subject to:  A*x <= b
    % with respect to:  A * x = b (equality constraint)
    % A*x <= b (inequality constraint)
    % solve QR problem
    % [matrix_result] = mpcCustomSolverCodeGen(single(H),single(f), single(-A_cons2), single(-b_cons2));
    matrix_result = single(zeros(Nc+1,1));
    matrix_result = MPC_Solver_QPhild(H,f',A_cons2,b_cons2);
    %% 4.计算前轮转角
    u_piao = matrix_result(1);
    U_k = single(kesi(3)) + u_piao;
    steer_cmd = ref_delta + U_k;
    %% 反算方向盘转角并转换为角度制
    if (steer_cmd>=0)
        steer_transmission_ratio = veh_params.left_steer_ratio;
    else
        steer_transmission_ratio = veh_params.right_steer_ratio;
    end
    steer_feedforward_temp  = ref_delta * single(57.3) * steer_transmission_ratio;%反算方向盘转角并转换为角度制deg
    steer_feedbackward_temp = U_k * single(57.3) * steer_transmission_ratio;%反算方向盘转角并转换为角度制deg
    steer_angle_cmd = steer_cmd * single(57.3) * steer_transmission_ratio;%反算方向盘转角并转换为角度制deg
    steer_angle_cmd_temp = steer_angle_cmd;%输出算法计算角度作为观测，最终请求角度会补偿转向不足。
    %% 5.限制期望前轮偏角
    % 5.1 根据横向加速度限制前轮转角
    if Veh_Speed < 1
        steer_limit = atan( Max_lateral_acceleration * veh_params.wheel_base /(Veh_Speed *Veh_Speed))* single(57.3) * steer_transmission_ratio; % 高速计算不准确，更改为下面特征车速计算方法
    else
        AckConst = min((single(1)+Veh_Speed*Veh_Speed/(veh_params.Vch*veh_params.Vch))*veh_params.wheel_base/max(single(1),Veh_Speed),single(32767));
        % PsiDtAckRaw = (SteerAngle/steer_transmission_ratio)/AckConst;
        steer_limit = ((Max_lateral_acceleration * AckConst)/Veh_Speed)* single(57.3) * steer_transmission_ratio;
    end
    %     steer_limit = atan( Max_lateral_acceleration * veh_params.wheel_base /(Veh_Speed *Veh_Speed)) * steer_transmission_ratio;
    steer_angle_cmd = min(steer_limit, max(-steer_limit,steer_angle_cmd));%方向盘角度制deg
    
    steer_angle_deg = steer_angle_cmd + CurrentSteerAngleOffset;
    steer_limit_temp = steer_limit;
    % 5.2 限制方向盘转速
    steer_angle = min(steer_angleK1 + TarSteerAngleSlope,max(steer_angleK1 - TarSteerAngleSlope,steer_angle_deg));
    
else
    U_k = single(0);
    matrix_result = single(zeros(6,1));
    steer_angle = SteerAngle;
    steer_angle_cmd_temp = single(0);
    steer_feedforward_temp = single(0);
    steer_feedbackward_temp = single(0);
    steer_limit_temp = single(0);
end
end

== matlab function PvtSubSys_LATC/LATC/LateralControl/LCS_Angle/Lateral_Control/MPC/Understeer_Offset_Calc/YOD_Ackman ==
  data: AckConst output; VxvRef input; Vch input; WheelBase input; AlpWheelAngle input; PsiDtAckK1 input single; PsiDtAck output
function [AckConst,PsiDtAck] = Ackman(VxvRef,Vch,WheelBase,AlpWheelAngle,PsiDtAckK1)
%#codegen
if VxvRef==uint8(0)%转换常数数据类型
    PsiDtAckRaw = single(0);%转换常数数据类型
    AckConst = single(1);%转换常数数据类型
else
    AckConst = min((single(1)+VxvRef*VxvRef/(Vch*Vch))*WheelBase/VxvRef,single(32767));%转换常数数据类型
    PsiDtAckRaw = AlpWheelAngle/AckConst;
end
PsiDtAck = (single(0.02/0.1))*(PsiDtAckRaw-PsiDtAckK1)+PsiDtAckK1;%转换常数数据类型

== matlab function PvtSubSys_LATC/LATC/LateralControl/LCS_Angle/Motion_Planning/FrenetTrajectory_Lateral/Subsystem1/MATLAB Function ==
  data: Forward_PreViewT input; VehSpd input; PreCurve output; C2 input; C3 input; PreCurve_Abs output
function [PreCurve,PreCurve_Abs]= PreView_Point_Curvature(Forward_PreViewT,VehSpd,C2,C3)
LookForwardDis = VehSpd * Forward_PreViewT;
PreCurve = 6*C3*LookForwardDis + 2*C2;
PreCurve_Abs = abs(PreCurve);
end

== matlab function PvtSubSys_LATC/LATC/LateralControl/LCS_Angle/Lateral_Control/MPC/TargetSteerAngleCalc/MATLAB Function ==
  data: c2 input; c1 input; c3 input; v input; PreCurve output; time input
function PreCurve = fcn(c2,c1,c3,v,time)
pdis = v*time;
% y1 = 3*c3*pdis^2 + 2*c2*pdis + c1;
PreCurve = 6*c3*pdis + 2*c2;
% r = y2/power((1+y1*y1),single(1.5));
end

== matlab function PvtSubSys_LATC/LATC/LateralControl/LCS_Angle/Motion_Planning/FrenetTrajectory_Lateral/Subsystem1/MATLAB Function1 ==
  data: Delaytime input uint16; Flg output uint8; Count output uint16; TarDangerLevel input uint8; TarDangerLevelK1 input uint8; FlgK1 input uint8; CountK1 input uint16
function [Flg,Count]= fcn(Delaytime,TarDangerLevel,TarDangerLevelK1,FlgK1,CountK1)
Count = min(CountK1 + uint16(1),Delaytime);
if Count == Delaytime
    Flg = uint8(0);
else
    Flg = FlgK1;
end
%%状态检测
if TarDangerLevel == uint8(1) && TarDangerLevelK1 == 0 %功能激活
    Count = uint16(0);
    Flg = uint8(1);  
end
end

== matlab function PvtSubSys_LATC/LATC/LateralControl/LCS_Angle/Motion_Planning/CartesianTrajectory_MPC/Subsystem/MATLAB Function ==
  data: c2 input; c1 input; c3 input; v input; PreCurve output; time input
function PreCurve = fcn(c2,c1,c3,v,time)
pdis = v*time;
% y1 = 3*c3*pdis^2 + 2*c2*pdis + c1;
PreCurve = 6*c3*pdis + 2*c2;
% r = y2/power((1+y1*y1),single(1.5));
end

== matlab function PvtSubSys_LATC/LATC/LateralControl/LCS_Angle/Lateral_Control/kinematics_MPC/Understeer&Offset_Calc/YOD_Ackman ==
  data: AckConst output; VxvRef input; Vch input; WheelBase input; AlpWheelAngle input; PsiDtAckK1 input single; PsiDtAck output
function [AckConst,PsiDtAck] = Ackman(VxvRef,Vch,WheelBase,AlpWheelAngle,PsiDtAckK1)
%#codegen
if VxvRef==uint8(0)%转换常数数据类型
    PsiDtAckRaw = single(0);%转换常数数据类型
    AckConst = single(1);%转换常数数据类型
else
    AckConst = min((single(1)+VxvRef*VxvRef/(Vch*Vch))*WheelBase/VxvRef,single(32767));%转换常数数据类型
    PsiDtAckRaw = AlpWheelAngle/AckConst;
end
PsiDtAck = (single(0.02/0.1))*(PsiDtAckRaw-PsiDtAckK1)+PsiDtAckK1;%转换常数数据类型

== matlab function PvtSubSys_LATC/LATC/LateralControl/LCS_Angle/Lateral_Control/kinematics_MPC/MATLAB Function ==
  data: PreviewX input; Delta_t output single; PreviewY input; VehSpd input
function Delta_t = fcn(PreviewX,PreviewY,VehSpd)
L = sqrt((PreviewX)^2 + (PreviewY)^2);
Delta_t = L/single(10*VehSpd);
end

== matlab function PvtSubSys_LATC/LATC/LateralControl/LCS_Angle/Lateral_Control/Trajectory_MPC/TargetSteerAngleCalc/MATLAB Function ==
  data: c2 input; c1 input; c3 input; v input; PreCurve output; time input
function PreCurve = fcn(c2,c1,c3,v,time)
pdis = v*time;
% y1 = 3*c3*pdis^2 + 2*c2*pdis + c1;
PreCurve = 6*c3*pdis + 2*c2;
% r = y2/power((1+y1*y1),single(1.5));
end

== matlab function PvtSubSys_LATC/LATC/LateralControl/LCS_Angle/Lateral_Control/Trajectory_MPC/TargetSteerAngleCalc/MATLAB Function3 ==
  data: delytime input uint16; TarDangerLevel input uint8; TarDangerLevelK1 input uint8; FLg output uint8; FLgK1 input uint8; CntK1 input uint16; Cnt output uint16
function [FLg,Cnt] = AngSlopeCalc(delytime,TarDangerLevel,TarDangerLevelK1,FLgK1,CntK1)

Cnt = min(CntK1 + uint16(1),delytime);
if Cnt== delytime
    FLg = uint8(0);
else
    FLg = FLgK1;
end
%FLg = FLgK1;
%% 换道开始检测
if TarDangerLevel==uint8(1) && TarDangerLevelK1==0  % NO function 2 LCK (TarDangerLevelK1==0)  %激活LCK
    Cnt =uint16(0);
    FLg = uint8(1);
end
%由LCK状态切换为Normal
if  TarDangerLevel==uint8(3) && (TarDangerLevelK1==uint8(1)||TarDangerLevelK1==uint8(2)) % LCK/IE 2 LC_Normal
    Cnt =uint16(0);
    FLg = uint8(2);
end
%由LCK状态切换为Eco
if  TarDangerLevel==uint8(7) && (TarDangerLevelK1==uint8(1)||TarDangerLevelK1==uint8(2)) % LCK/IE 2 LC_Eco
    Cnt =uint16(0);
    FLg = uint8(3);
end
%由LCK状态切换为Sport
if  TarDangerLevel==uint8(8) && (TarDangerLevelK1==uint8(1)||TarDangerLevelK1==uint8(2)) % LCK/IE 2 LC_sport
    Cnt =uint16(0);
    FLg = uint8(4);
end
if  TarDangerLevel==uint8(6) && (TarDangerLevelK1==uint8(1)||TarDangerLevelK1==uint8(2)) % LCK/IE 2 ESS 后期添加配和ESS Slope 一起调试
    Cnt =uint16(0);
    FLg = uint8(5);
end
%% 换道完成检测，主要时为了解决换道完成后切换到LCK后Angleslope太小导致超调，检测到换道完成后延时一段时间保持一个大斜率。
if  (TarDangerLevel==uint8(1)||TarDangerLevel==uint8(2)) && (TarDangerLevelK1==uint8(3)) % LCK/IE 2 LC_Normal Complete
    Cnt =uint16(0);
    FLg = uint8(6);
end
if  (TarDangerLevel==uint8(1)||TarDangerLevel==uint8(2)) && (TarDangerLevelK1==uint8(7)) % LCK/IE 2 LC_Eco Complete
    Cnt =uint16(0);
    FLg = uint8(7);
end
if  (TarDangerLevel==uint8(1)||TarDangerLevel==uint8(2)) && (TarDangerLevelK1==uint8(8)) % LCK/IE 2 LC_sport Complete
    Cnt =uint16(0);
    FLg = uint8(8);
end

== matlab function PvtSubSys_LATC/LATC/LateralControl/LCS_Angle/Lateral_Control/Trajectory_MPC/TargetSteerAngleCalc/TargetSteerAngleCalc ==
  data: LineValid input boolean size=1; TarSteerAngle output single size=1; TarSteerAngleEnd output single size=1; Xn output single; Yn output single; Yawn output single; Num output uint8 size=1; J output single; Jr1 output single; Jq output single; vxvRef input single size=1; SteerAngle input single size=1; Charspd input single size=1; WheelBase input single size=1; SteerRatio input single size=1; tDeltaEPS input single size=1; PreDis input single size=1; TarSteerAngleSlope input single size=1; R1 input single size=1; Q input single size=1; TarSteerAngleK1 input single size=1; ADDANGLE output; CurrentSteerAngleOffset input single; SteerAngleOffset_deg input; LCS_PlanX input; LCS_PlanY input
function [TarSteerAngle,TarSteerAngleEnd,Xn,Yn,Yawn,Num,J,Jr1,Jq,ADDANGLE] = ...
    TargetSteerAngleCalc(LineValid,vxvRef,SteerAngle,Charspd,WheelBase,SteerRatio,tDeltaEPS,PreDis,TarSteerAngleSlope,R1,Q,...
    TarSteerAngleK1,CurrentSteerAngleOffset,SteerAngleOffset_deg,...
    LCS_PlanX,LCS_PlanY)

StrToWhlFac = 57.3*SteerRatio;  %弧度转换角度
SteerAngleSpdLimit = single(TarSteerAngleSlope*50);  %方向盘转动变化率限制(°/s)
dxOffset = single(2.1);  %车辆前轴的距离

Delta = single([-45,-40, -35, -30,-27,-24,-21, -18,-15, -12,-10, -8,-6,-5,...
         -4.5,-4,-3.5,-3, -2.5,-2, -1.5, -1,-0.5, 0,0.5, 1, 1.5, 2,...
         2.5,3,3.5,4,4.5, 5 ,6 ,8, 10,12,15,18,21,24,27,30,35,40,45]);

J = single(zeros(length(Delta),1));
Jr1 = single(zeros(length(Delta),1));
Jq = single(zeros(length(Delta),1));
vRef = max(vxvRef,single(0.1));

if LineValid
    % 20 Calculate Cycle
    Step_Dis = PreDis/single(49);                   %将规划轨迹均分50等份
    SteerAngleMa = single(zeros(length(Delta),20)); %方向盘转角矩阵
    YawMa = single(zeros(length(Delta),20));        %车身朝向角
    YiMa = single(zeros(length(Delta),20));         %横坐标
    XiMa = single(zeros(length(Delta),20));         %纵坐标
    Traj_Valid = true(length(Delta),1);
    Jmin =single(-1);
    Num = uint8(0);

    for k = uint8(1:1:length(Delta))
        SteerAngleRaw = SteerAngle + Delta(k);       %方向盘实际有效转角+预期方向盘增量
        Step_T = Step_Dis/vRef;                      %行驶完每一份规划轨迹所用的时间（预测步长）
        %% 推算每条轨迹下每个轨迹点处方向盘转角
        SteerAngleMa(k,1) =  TarSteerAngleK1;        %计算31条轨迹起始位置的方向盘转角
        for i = 2:20                                 %每条轨迹的20个轨迹点之间的预测步长选择（变步长）
            if i<=5
                Delta_T = Step_T * single((i-1));
            elseif i<=10
                Delta_T = 4*Step_T + 2*Step_T*single((i-5));
            elseif i<=15
                Delta_T = 14*Step_T + 3*Step_T*single((i-10));
            else
                Delta_T = 29*Step_T + 4*Step_T*single((i-15));
            end
            
            if SteerAngleRaw > TarSteerAngleK1    %判断转向方向  方向盘转角左正右负  
                SteerAngleMa(k,i) = TarSteerAngleK1 + Delta_T*SteerAngleSpdLimit;%计算每条轨迹下的20个方向盘转角
                                                                                  %不用Delta_T*(i-1)*SteerAngleSpdLimit的原因是：这种写法与前面的50步冲突
                SteerAngleMa(k,i) = min(SteerAngleMa(k,i),SteerAngleRaw);% 
            else
                SteerAngleMa(k,i) = TarSteerAngleK1 - Delta_T*SteerAngleSpdLimit;
                SteerAngleMa(k,i) = max(SteerAngleMa(k,i),SteerAngleRaw);
            end
        end
        %% 计算每条轨迹起始点(第一个点)的坐标及车身朝向角
        if vRef<1
            YawMa(k,1) = tDeltaEPS*vRef*tan((SteerAngle)/StrToWhlFac)/WheelBase; % 计算每一条推算轨迹起始位置的车身朝向角（单位：rad）
        else
            AckConst = min((single(1)+vRef*vRef/(Charspd*Charspd))*WheelBase/max(single(1),vRef),single(32767));          %计算稳态横摆角速度增益 （单位：s）
            YawMa(k,1) = tDeltaEPS*(SteerAngle)/(AckConst*StrToWhlFac);     % 计算每一条推算轨迹起始位置的车身朝向角(角度)
        end
        XiMa(k,1) = tDeltaEPS*vRef*cos(YawMa(k,1));%推算第一步纵向坐标
        YiMa(k,1) = tDeltaEPS*vRef*sin(YawMa(k,1));%推算第一步横向坐标
        %% 转向cost
        uDelta = SteerAngleMa(k,3) - SteerAngleMa(k,1);
        %%
        for i=1:19
            if i<=5
                StepDisFac = single(1);
            elseif i<=10
                StepDisFac = single(2);
            elseif i<=15
                StepDisFac = single(3);
            else
                StepDisFac = single(4);
            end
            if vRef<1
                t_kap = tan(SteerAngleMa(k,i)/StrToWhlFac)/WheelBase;  %计算每一个方向盘转角下对应的曲率
                YawMa(k,i+1) = YawMa(k,i) + StepDisFac*Step_Dis*t_kap;  %计算每一条推算轨迹除起始位置的车身朝向角
            else
                T_Step = StepDisFac*Step_Dis/vRef;
                AckConst = min((single(1)+vRef*vRef/(Charspd*Charspd))*WheelBase/vRef,single(32767));
                YawRate = SteerAngleMa(k,i)/(AckConst*StrToWhlFac); % 横摆角速度
                YawMa(k,i+1) = YawMa(k,i) + YawRate*T_Step;         % 每一步结束后的车辆朝向角
            end
            
            if (YawMa(k,i+1)>single(1.2))||(YawMa(k,i+1)<single(-1.2)) %筛选推算轨迹(如果朝向角度相对于参考线误差太大直接舍去)
                Traj_Valid(k) = false;
            else
                XiMa(k,i+1) = XiMa(k,i) + StepDisFac*Step_Dis *cos(0.5*(YawMa(k,i)+YawMa(k,i+1))); %计算每一个推算点的纵向坐标 XiMa(k,i+1) = XiMa(k,i) + StepDisFac*Step_Dis *cos((YawMa(k,i));
                YiMa(k,i+1) = YiMa(k,i) + StepDisFac*Step_Dis *sin(0.5*(YawMa(k,i)+YawMa(k,i+1))); %计算每一个推算点的横向坐标
            end
        end
        if Traj_Valid(k) == true
            % 推算车辆前轴中心点的位置坐标
            for i = single(1):single(1):single(20)
                XiMa(k,i) = XiMa(k,i) + dxOffset*cos(YawMa(k,i));
                YiMa(k,i) = YiMa(k,i) + dxOffset*sin(YawMa(k,i));
            end
            % 计算损失量
            PlanYi = single(zeros(1,20));
            PlanYi = interp1(LCS_PlanX',LCS_PlanY',XiMa(k,1:20),'linear');
            Jr1(k) = R1*sum(((YiMa(k,1:20) - PlanYi(k,1:20)).^2));      %规划点与控制点之间的横向误差最小（说明两个轨迹贴合程度较高）
            J(k) = J(k) + Jr1(k);
        end   
        % 第K步的损失量
        Jq(k) = Q*uDelta^2;
        J(k) = J(k) + Jq(k);
        % 筛选出最小损失的轨迹
        if Jmin<0
            Jmin = J(k);
            Num = k;
        else
            if J(k)<=Jmin
                Jmin = J(k);
                Num = k;
            end
        end
    end
    TarSteerAngleEnd = SteerAngle + Delta(Num); %算法实际算出的最终方向盘转角(应该是当前的还是上一帧的存在模糊点)   
    TarSteerAngle = min(TarSteerAngleK1 + TarSteerAngleSlope,max(TarSteerAngleK1 - TarSteerAngleSlope,TarSteerAngleEnd)); 
   % 为舒适性，方向盘转角不能一下按照算法计算出来的角度执行，所以要对方向盘转角进行限制
    Xn = XiMa(Num,1:20);
    Yn = YiMa(Num,1:20);
    Yawn = YawMa(Num,1:20);
    ADDANGLE=Delta(Num);
else
    TarSteerAngle = SteerAngle+SteerAngleOffset_deg-CurrentSteerAngleOffset;
    TarSteerAngleEnd = SteerAngle;
    Xn = single(zeros(1,20));
    Yn = single(zeros(1,20));
    Yawn = single(zeros(1,20));
    Num = uint8(0);
    ADDANGLE = single(zeros(1,1));
end
end

== matlab function PvtSubSys_LATC/LATC/LateralControl/LCS_Angle/Lateral_Control/Trajectory_MPC/Understeer_Offset_Calc/YOD_Ackman ==
  data: AckConst output; VxvRef input; Vch input; WheelBase input; AlpWheelAngle input; PsiDtAckK1 input single; PsiDtAck output
function [AckConst,PsiDtAck] = Ackman(VxvRef,Vch,WheelBase,AlpWheelAngle,PsiDtAckK1)
%#codegen
if VxvRef==uint8(0)%转换常数数据类型
    PsiDtAckRaw = single(0);%转换常数数据类型
    AckConst = single(1);%转换常数数据类型
else
    AckConst = min((single(1)+VxvRef*VxvRef/(Vch*Vch))*WheelBase/VxvRef,single(32767));%转换常数数据类型
    PsiDtAckRaw = AlpWheelAngle/AckConst;
end
PsiDtAck = (single(0.02/0.1))*(PsiDtAckRaw-PsiDtAckK1)+PsiDtAckK1;%转换常数数据类型
